simulink model "nms_3Dmodel"  (Simulink 9.3)
settings: Solver=ode15s  StartTime=0.0  StopTime=20  FixedStep=1e-3  RelTol=1e-3  AbsTol=1e-4  EnableMultiTasking=on
InitFcn:
  | runScripts;
undefined symbols (not defined in the file or in its folder): ankle_height, c, c_jointstop, CtrlPar_FP, CtrlPar_FP_R, CtrlPar_LL, CtrlPar_St, CtrlPar_St_R, CtrlPar_Sw, CtrlPar_Sw_R, CtrlPar_theta0, CtrlPar_Tr, CtrlPar_Tr_R, D12_F, D12_S, D12_T, D12z_T, D13_F, D1G_F, D1G_HAT, D1G_S, D1G_T, D1Gy_F, d_fBall, d_fHeel, DeltaThRef, dt, eref, FmaxBFSH, FmaxGAS, FmaxGLU, FmaxHAB, FmaxHAD, FmaxHAM, FmaxHFL, FmaxRF, FmaxSOL, FmaxTA, FmaxVAS, In_F, In_HAT, In_S, In_T, init_a_tgt, init_a_tgtR, Inx_F, Inx_HAT, Inx_S, Inx_T, Iny_F, Iny_HAT, Iny_S, Iny_T, K, k_gn, k_gt, k_pressure, leg_l, LongDelay, LongLoopDelay ... (+137)
libraries: mblibv1 x88, simulink x44, simulink_extras x38
(part 3 of 13)

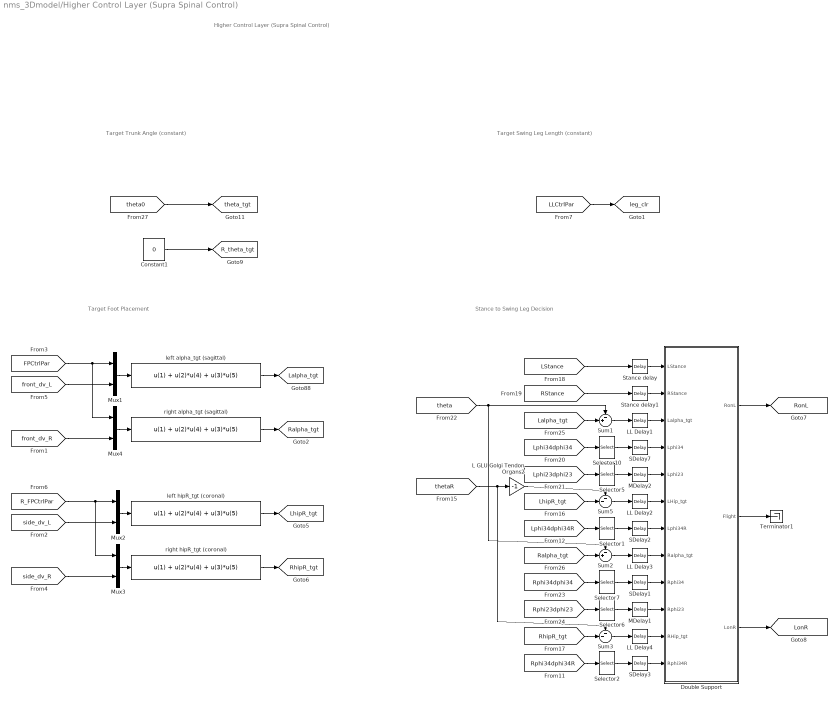
== system nms_3Dmodel/Higher Control Layer (Supra Spinal Control) ==
  note: Target Foot Placement
  note: Target Swing Leg Length
      | (constant)
  note: Stance to Swing Leg Decision
  note: Target Trunk Angle
      | (constant)
  note: Higher Control Layer
      | (Supra Spinal Control)
  Constant1 : Constant  Value=0
  Double Support : Subsystem
  L GLU Golgi Tendon Organs2 : Gain  Gain=-1
  LL Delay1 : TransportDelay  DelayTime=LongLoopDelay/2  InitialOutput=init_a_tgt
  LL Delay2 : TransportDelay  DelayTime=LongLoopDelay/2
  LL Delay3 : TransportDelay  DelayTime=LongLoopDelay/2  InitialOutput=init_a_tgt
  LL Delay4 : TransportDelay  DelayTime=LongLoopDelay/2
  MDelay1 : TransportDelay  DelayTime=MidDelay
  MDelay2 : TransportDelay  DelayTime=MidDelay
  Mux{1..4} (4 alike) : Mux  Inputs=2
  SDelay{1..3,7} (4 alike) : TransportDelay  DelayTime=ShortDelay
  Selector{1..2,5..7,10} (6 alike) : Selector  InputPortWidth=2  IndexOptions=Index vector (dialog)  Indices=1  OutputSizes=1
  Stance delay : TransportDelay  DelayTime=MidDelay
  Stance delay1 : TransportDelay  DelayTime=MidDelay
  Sum1 : Sum  Inputs=-+|
  Sum2 : Sum  Inputs=-+|
  Sum3 : Sum  Inputs=--|
  Sum5 : Sum  Inputs=--|
  Terminator1 : Terminator
  left alpha_tgt (sagittal) : Fcn  Expr=u(1) + u(2)*u(4) + u(3)*u(5)
  left hipR_tgt (coronal) : Fcn  Expr=u(1) + u(2)*u(4) + u(3)*u(5)
  right alpha_tgt (sagittal) : Fcn  Expr=u(1) + u(2)*u(4) + u(3)*u(5)
  right hipR_tgt (coronal) : Fcn  Expr=u(1) + u(2)*u(4) + u(3)*u(5)
  tag scope: Lalpha_tgt=global, LhipR_tgt=global, LonR=global, R_theta_tgt=global, Ralpha_tgt=global, RhipR_tgt=global, RonL=global, leg_clr=global, theta_tgt=global
  wires:
  left alpha_tgt (sagittal)/1 -> [Lalpha_tgt]
  right alpha_tgt (sagittal)/1 -> [Ralpha_tgt]
  left hipR_tgt (coronal)/1 -> [LhipR_tgt]
  right hipR_tgt (coronal)/1 -> [RhipR_tgt]
  [LLCtrlPar] -> [leg_clr]
  [Lphi34dphi34] -> Selector10/1
  [Lphi23dphi23] -> Selector5/1
  Selector10/1 -> SDelay7/1
  Selector5/1 -> MDelay2/1
  [Rphi34dphi34] -> Selector7/1
  [Rphi23dphi23] -> Selector6/1
  Selector7/1 -> SDelay1/1
  Selector6/1 -> MDelay1/1
  Double Support/3(LonR) -> [LonR]
  Stance delay/1 -> Double Support/1(LStance)
  Stance delay1/1 -> Double Support/2(RStance)
  Double Support/1(RonL) -> [RonL]
  [LStance] -> Stance delay/1
  [RStance] -> Stance delay1/1
  Double Support/2(Flight) -> Terminator1/1
  LL Delay1/1 -> Double Support/3(Lalpha_tgt)
  LL Delay3/1 -> Double Support/8(Ralpha_tgt)
  SDelay7/1 -> Double Support/4(Lphi34)
  SDelay1/1 -> Double Support/9(Rphi34)
  MDelay2/1 -> Double Support/5(Lphi23)
  MDelay1/1 -> Double Support/10(Rphi23)
  Sum1/1 -> LL Delay1/1
  [Lalpha_tgt] -> Sum1/2
  [theta] -> Sum1/1, Sum2/1
  [Ralpha_tgt] -> Sum2/2
  Sum2/1 -> LL Delay3/1
  [Lphi34dphi34R] -> Selector1/1
  Selector1/1 -> SDelay2/1
  SDelay2/1 -> Double Support/7(Lphi34R)
  LL Delay2/1 -> Double Support/6(LHip_tgt)
  Sum5/1 -> LL Delay2/1
  [LhipR_tgt] -> Sum5/2
  [thetaR] -> L GLU Golgi Tendon Organs2/1, Sum3/1
  L GLU Golgi Tendon Organs2/1 -> Sum5/1
  [Rphi34dphi34R] -> Selector2/1
  Selector2/1 -> SDelay3/1
  SDelay3/1 -> Double Support/12(Rphi34R)
  LL Delay4/1 -> Double Support/11(RHip_tgt)
  Sum3/1 -> LL Delay4/1
  [RhipR_tgt] -> Sum3/2
  [theta0] -> [theta_tgt]
  Constant1/1 -> [R_theta_tgt]
  Mux1/1 -> left alpha_tgt (sagittal)/1
  [FPCtrlPar] -> Mux4/1, Mux1/1
  [front_dv_L] -> Mux1/2
  Mux4/1 -> right alpha_tgt (sagittal)/1
  [front_dv_R] -> Mux4/2
  Mux2/1 -> left hipR_tgt (coronal)/1
  Mux3/1 -> right hipR_tgt (coronal)/1
  [R_FPCtrlPar] -> Mux3/1, Mux2/1
  [side_dv_L] -> Mux2/2
  [side_dv_R] -> Mux3/2

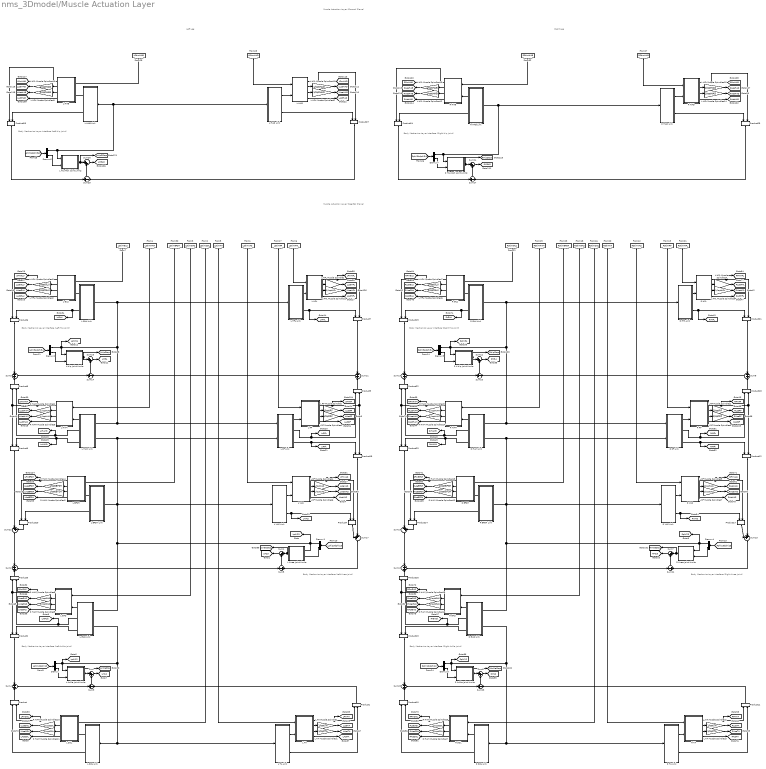
== system nms_3Dmodel/Muscle Actuation Layer ==
  note: Muscle Actuation Layer
      | (Sagittal Plane)
  note: Body Mechanics Layer
      | Interface (Left Hip Joint)
  note: Body Mechanics Layer
      | Interface (Left Knee Joint)
  note: Body Mechanics Layer
      | Interface (Left Ankle Joint)
  note: Body Mechanics Layer
      | Interface (Right Hip Joint)
  note: Body Mechanics Layer
      | Interface (Right Knee Joint)
  note: Body Mechanics Layer
      | Interface (Right Ankle Joint)
  note: Left Leg
  note: Body Mechanics Layer
      | Interface (Left Hip Joint)
  note: Body Mechanics Layer
      | Interface (Right Hip Joint)
  note: Right Leg
  note: Muscle Actuation Layer
      | (Coronal Plane)
  Demux{,1..7} (8 alike) : Demux  Outputs=2
  L Ankle Joint Limits : Subsystem
  L BFSH : Subsystem
  L BFSH Link : Subsystem
  L GAS : Subsystem
  L GAS Link : Subsystem
  L GLU : Subsystem
  L GLU Link : Subsystem
  L HAB : Subsystem
  L HAB Link : Subsystem
  L HAD : Subsystem
  L HAD Link : Subsystem
  L HAM : Subsystem
  L HAM Link : Subsystem
  L HFL : Subsystem
  L HFL Muscle Spindles{,1,4..5} (4 alike) : Gain  Gain=1/loptHFL
  L HFL Muscle Spindles{9..10,12..13} (4 alike) : Gain  Gain=1/loptHAB
  L HFL Muscle Spindles{8,11,14..15} (4 alike) : Gain  Gain=1/loptHAD
  L HFL Muscle Spindles{2..3,6..7} (4 alike) : Gain  Gain=1/loptGLU
  L HFL Link : Subsystem
  L Hip Joint Limits : Subsystem
  L Hip Roll Joint Limits : Subsystem
  L Knee Joint Limits : Subsystem
  L RF : Subsystem
  L RF Muscle Spindles{,1..3} (4 alike) : Gain  Gain=1/loptRF
  L RF Muscle Spindles{4..7} (4 alike) : Gain  Gain=1/loptVAS
  L RF Link : Subsystem
  L SOL : Subsystem
  L SOL Link : Subsystem
  L TA : Subsystem
  L TA Muscle Spindles{,1..3} (4 alike) : Gain  Gain=1/loptTA
  L TA Link : Subsystem
  L VAS : Subsystem
  L VAS Link : Subsystem
  Product{,1..27} (28 alike) : Product  RndMeth=Zero
  R Ankle Joint Limits : Subsystem
  R BFSH : Subsystem
  R BFSH Link : Subsystem
  R GAS : Subsystem
  R GAS Link : Subsystem
  R GLU : Subsystem
  R GLU Link : Subsystem
  R HAB : Subsystem
  R HAB Link : Subsystem
  R HAD : Subsystem
  R HAD Link : Subsystem
  R HAM : Subsystem
  R HAM Muscle Spindles{1,3,6,14} (4 alike) : Gain  Gain=1/loptHAM
  R HAM Muscle Spindles{5,7,10..11} (4 alike) : Gain  Gain=1/loptSOL
  R HAM Muscle Spindles{2,4,12..13} (4 alike) : Gain  Gain=1/loptBFSH
  R HAM Muscle Spindles{8..9,15..16} (4 alike) : Gain  Gain=1/loptGAS
  R HAM Link : Subsystem
  R HFL : Subsystem
  R HFL Link : Subsystem
  R Hip Roll Joint Limits : Subsystem
  R Knee Joint Limits : Subsystem
  R L Hip Joint Limits : Subsystem
  R RF : Subsystem
  R RF Link : Subsystem
  R SOL : Subsystem
  R SOL Link : Subsystem
  R TA : Subsystem
  R TA Link : Subsystem
  R VAS : Subsystem
  R VAS Link : Subsystem
  Sum{,1,6..7,12,16,18,22,24,26} (10 alike) : Sum  Inputs=|++
  Sum{9..10,14,23,25,27} (6 alike) : Sum  Inputs=+-
  Sum{2..4,8,11,15,19..20} (8 alike) : Sum
  Sum13 : Sum  Inputs=++|
  Sum17 : Sum  Inputs=++|
  Sum21 : Sum  Inputs=-+
  Sum5 : Sum  Inputs=-+
  tag scope: LActBFSH=global, LActGAS=global, LActGLU=global, LActHAB=global, LActHAD=global, LActHAM=global, LActHFL=global, LActRF=global, LActSOL=global, LActTA=global, LActVAS=global, LAnkleStop=global, LFmBFSH=global, LFmGAS=global, LFmGLU=global, LFmHAB=global, LFmHAD=global, LFmHAM=global, LFmHFL=global, LFmRF=global, LFmSOL=global, LFmTA=global, LFmVAS=global, LHipRStop=global, LHipStop=global, LKneeStop=global, LLceBFSH=global, LLceGAS=global, LLceGLU=global, LLceHAB=global, LLceHAD=global, LLceHAM=global, LLceHFL=global, LLceRF=global, LLceSOL=global, LLceTA=global, LLceVAS=global, LM12=global, LM23=global, LM34=global, LM34R=global, LVceBFSH=global, LVceGAS=global, LVceGLU=global, LVceHAB=global, LVceHAD=global, LVceHAM=global, LVceHFL=global, LVceRF=global, LVceSOL=global, LVceTA=global, LVceVAS=global, Lphi12=global, Lphi23=global, Lphi34=global, LrGASk=global, LrGLU=global, LrHAMh=global, LrHAMk=global, LrHFL=global, LrRFh=global, LrRFk=global, LrVAS=global, RActBFSH=global, RActGAS=global, RActGLU=global, RActHAB=global, RActHAD=global, RActHAM=global, RActHFL=global, RActRF=global, RActSOL=global, RActTA=global, RActVAS=global, RAnkleStop=global, RFmBFSH=global, RFmGAS=global, RFmGLU=global, RFmHAB=global, RFmHAD=global, RFmHAM=global, RFmHFL=global, RFmRF=global, RFmSOL=global, RFmTA=global, RFmVAS=global, RHipStop=global, RHipStopR=global, RKneeStop=global, RLceBFSH=global, RLceGAS=global, RLceGLU=global, RLceHAB=global, RLceHAD=global, RLceHAM=global, RLceHFL=global, RLceRF=global, RLceSOL=global, RLceTA=global, RLceVAS=global, RM12=global, RM23=global, RM34=global, RM34R=global, RVceBFSH=global, RVceGAS=global, RVceGLU=global, RVceHAB=global, RVceHAD=global, RVceHAM=global, RVceHFL=global, RVceRF=global, RVceSOL=global, RVceTA=global, RVceVAS=global, Rphi12=global, Rphi23=global, Rphi34=global, RrGASk=global, RrGLU=global, RrHAMh=global, RrHAMk=global, RrHFL=global, RrRFh=global, RrRFk=global, RrVAS=global
  wires:
  Demux1/1 -> L Knee Joint Limits/1(phi [rad]), L VAS Link/1(phi23 [rad]), L RF Link/2(phi23 [rad]), L HAM Link/2(phi23 [rad]), L BFSH Link/1(phi23 [rad]), L GAS Link/1(phi23 [rad]), [Lphi23]
  L SOL/1(Fmtc) -> Product/2, [LFmSOL]
  L TA/2(Lce) -> L TA Muscle Spindles/1
  L TA/4(A) -> [LActTA]
  L GAS/1(Fmtc) -> Product2/1, Product3/1, [LFmGAS]
  Demux/1 -> L SOL Link/1(phi12 [rad]), L TA Link/1(phi12 [rad]), L GAS Link/2(phi12 [rad]), L Ankle Joint Limits/1(phi [rad]), [Lphi12]
  [LStimTA] -> L TA/1(STIM)
  [LStimSOL] -> L SOL/1(STIM)
  [LStimHAM] -> L HAM/1(STIM)
  L HAM/1(Fmtc) -> Product9/1, Product8/1, [LFmHAM]
  L HAM/2(Lce) -> R HAM Muscle Spindles1/1
  L HFL/1(Fmtc) -> Product7/2, [LFmHFL]
  L HFL/2(Lce) -> L HFL Muscle Spindles/1
  [LStimHFL] -> L HFL/1(STIM)
  L GLU/1(Fmtc) -> Product6/1, [LFmGLU]
  [LStimGLU] -> L GLU/1(STIM)
  Sum16/1 -> [LM34]
  Demux/2 -> L Ankle Joint Limits/2(dphi [rad/s])
  Sum9/1 -> Sum/2
  Demux1/2 -> L Knee Joint Limits/2(dphi [rad/s])
  L SOL Link/1(lmtc [m]) -> L SOL/2(lmtc [m])
  L TA Link/1(lmtc [m]) -> L TA/2(lmtc [m])
  L GAS Link/3(lever12 [m]) -> Product2/2
  L GAS Link/2(lever23 [m]) -> Product3/2, [LrGASk]
  [LStimGAS] -> L GAS/1(STIM)
  L GAS Link/1(lmtu [m]) -> L GAS/2(lmtc [m])
  L VAS Link/1(lmtu [m]) -> L VAS/2(lmtc [m])
  L HAM Link/1(lmtu [m]) -> L HAM/2(lmtc [m])
  L HAM Link/2(lever34 [m]) -> Product8/2, [LrHAMh]
  L HAM Link/3(lever23 [m]) -> Product9/2, [LrHAMk]
  Product3/1 -> Sum2/2
  Sum3/1 -> Sum14/1
  Sum4/1 -> Sum9/1
  [Lphi12dphi12] -> Demux/1
  [Lphi23dphi23] -> Demux1/1
  [Lphi34dphi34] -> Demux2/1
  Demux2/1 -> L Hip Joint Limits/1(phi [rad]), L HFL Link/1(phi34 [rad]), L GLU Link/1(phi34 [rad]), L RF Link/1(phi34 [rad]), L HAM Link/1(phi34 [rad]), [Lphi34]
  L SOL Link/2(lever [m]) -> Product/1
  Product/1 -> Sum4/2
  Product2/1 -> Sum4/1
  L TA Link/2(lever [m]) -> Product1/2
  Product1/1 -> Sum9/2
  L Ankle Joint Limits/1(M_stop [Nm]) -> Sum/1, [LAnkleStop]
  Sum/1 -> [LM12]
  L SOL/4(A) -> [LActSOL]
  L GAS/4(A) -> [LActGAS]
  L VAS/4(A) -> [LActVAS]
  L VAS/1(Fmtc) -> Product4/2, [LFmVAS]
  Sum1/1 -> [LM23]
  L Knee Joint Limits/1(M_stop [Nm]) -> Sum1/1, [LKneeStop]
  Sum5/1 -> Sum1/2
  L VAS Link/2(lever [m]) -> [LrVAS], Product4/1
  Sum2/1 -> Sum5/1
  L HAM/4(A) -> [LActHAM]
  Product8/1 -> Sum3/2
  Product6/1 -> Sum3/1
  L GLU Link/1(lmtu [m]) -> L GLU/2(lmtc [m])
  L GLU Link/2(lever [m]) -> Product6/2, [LrGLU]
  L GLU/4(A) -> [LActGLU]
  Demux2/2 -> L Hip Joint Limits/2(dphi [rad/s])
  L Hip Joint Limits/1(M_stop [Nm]) -> Sum16/1, [LHipStop]
  Sum14/1 -> Sum16/2
  L HFL Link/1(lmtu [m]) -> L HFL/2(lmtc [m])
  L HFL/4(A) -> [LActHFL]
  L HFL Link/2(lever [m]) -> Product7/1, [LrHFL]
  [LStimVAS] -> L VAS/1(STIM)
  L GLU/2(Lce) -> L HFL Muscle Spindles3/1
  L GLU/3(Vce) -> L HFL Muscle Spindles2/1
  L HAM/3(Vce) -> R HAM Muscle Spindles6/1
  L GAS/3(Vce) -> R HAM Muscle Spindles9/1
  L GAS/2(Lce) -> R HAM Muscle Spindles8/1
  L SOL/2(Lce) -> R HAM Muscle Spindles10/1
  L SOL/3(Vce) -> R HAM Muscle Spindles11/1
  L TA/3(Vce) -> L TA Muscle Spindles1/1
  L VAS/3(Vce) -> L RF Muscle Spindles6/1
  L VAS/2(Lce) -> L RF Muscle Spindles4/1
  L HFL/3(Vce) -> L HFL Muscle Spindles1/1
  L RF/4(A) -> [LActRF]
  L RF/3(Vce) -> L RF Muscle Spindles2/1
  L RF/2(Lce) -> L RF Muscle Spindles/1
  L RF Link/1(lmtu [m]) -> L RF/2(lmtc [m])
  L RF Link/2(lever34 [m]) -> Product5/1, [LrRFh]
  L RF Link/3(lever23 [m]) -> Product15/1, [LrRFk]
  [LStimRF] -> L RF/1(STIM)
  Product7/1 -> Sum11/1
  Product5/1 -> Sum11/2
  Product15/1 -> Sum17/2
  Sum17/1 -> Sum5/2
  Product4/1 -> Sum17/1
  [LStimBFSH] -> L BFSH/1(STIM)
  L BFSH Link/1(lmtu [m]) -> L BFSH/2(lmtc [m])
  L BFSH Link/2(lever [m]) -> Product20/2
  L BFSH/4(A) -> [LActBFSH]
  L BFSH/2(Lce) -> R HAM Muscle Spindles4/1
  L BFSH/3(Vce) -> R HAM Muscle Spindles2/1
  Product20/1 -> Sum22/2
  Sum22/1 -> Sum2/1
  Product9/1 -> Sum22/1
  L HFL Muscle Spindles1/1 -> [LVceHFL]
  L HFL Muscle Spindles2/1 -> [LVceGLU]
  L HFL Muscle Spindles3/1 -> [LLceGLU]
  L RF Muscle Spindles6/1 -> [LVceVAS]
  L RF/1(Fmtc) -> Product5/2, Product15/2, [LFmRF]
  L BFSH/1(Fmtc) -> Product20/1, [LFmBFSH]
  R HAM Muscle Spindles8/1 -> [LLceGAS]
  R HAM Muscle Spindles9/1 -> [LVceGAS]
  R HAM Muscle Spindles10/1 -> [LLceSOL]
  R HAM Muscle Spindles11/1 -> [LVceSOL]
  L TA/1(Fmtc) -> Product1/1, [LFmTA]
  L TA Muscle Spindles1/1 -> [LVceTA]
  L HFL Muscle Spindles/1 -> [LLceHFL]
  R HAM Muscle Spindles1/1 -> [LLceHAM]
  R HAM Muscle Spindles6/1 -> [LVceHAM]
  L RF Muscle Spindles/1 -> [LLceRF]
  L RF Muscle Spindles2/1 -> [LVceRF]
  R HAM Muscle Spindles4/1 -> [LLceBFSH]
  R HAM Muscle Spindles2/1 -> [LVceBFSH]
  L RF Muscle Spindles4/1 -> [LLceVAS]
  L TA Muscle Spindles/1 -> [LLceTA]
  Demux4/1 -> R Knee Joint Limits/1(phi [rad]), R VAS Link/1(phi23 [rad]), R RF Link/2(phi23 [rad]), R HAM Link/2(phi23 [rad]), R BFSH Link/1(phi23 [rad]), R GAS Link/1(phi23 [rad]), [Rphi23]
  R SOL/1(Fmtc) -> Product10/2, [RFmSOL]
  R TA/2(Lce) -> L TA Muscle Spindles2/1
  R TA/4(A) -> [RActTA]
  R GAS/1(Fmtc) -> Product13/1, Product16/1, [RFmGAS]
  Demux3/1 -> R SOL Link/1(phi12 [rad]), R TA Link/1(phi12 [rad]), R GAS Link/2(phi12 [rad]), R Ankle Joint Limits/1(phi [rad]), [Rphi12]
  [RStimTA] -> R TA/1(STIM)
  [RStimSOL] -> R SOL/1(STIM)
  [RStimHAM] -> R HAM/1(STIM)
  R HAM/1(Fmtc) -> Product23/1, Product22/1, [RFmHAM]
  R HAM/2(Lce) -> R HAM Muscle Spindles3/1
  R HFL/1(Fmtc) -> Product21/2, [RFmHFL]
  R HFL/2(Lce) -> L HFL Muscle Spindles4/1
  [RStimHFL] -> R HFL/1(STIM)
  R GLU/1(Fmtc) -> Product19/1, [RFmGLU]
  [RStimGLU] -> R GLU/1(STIM)
  Sum12/1 -> [RM34]
  Demux3/2 -> R Ankle Joint Limits/2(dphi [rad/s])
  Sum23/1 -> Sum6/2
  Demux4/2 -> R Knee Joint Limits/2(dphi [rad/s])
  R SOL Link/1(lmtc [m]) -> R SOL/2(lmtc [m])
  R TA Link/1(lmtc [m]) -> R TA/2(lmtc [m])
  R GAS Link/3(lever12 [m]) -> Product13/2
  R GAS Link/2(lever23 [m]) -> Product16/2, [RrGASk]
  [RStimGAS] -> R GAS/1(STIM)
  R GAS Link/1(lmtu [m]) -> R GAS/2(lmtc [m])
  R VAS Link/1(lmtu [m]) -> R VAS/2(lmtc [m])
  R HAM Link/1(lmtu [m]) -> R HAM/2(lmtc [m])
  R HAM Link/2(lever34 [m]) -> Product22/2, [RrHAMh]
  R HAM Link/3(lever23 [m]) -> Product23/2, [RrHAMk]
  Product16/1 -> Sum15/2
  Sum19/1 -> Sum10/1
  Sum20/1 -> Sum23/1
  [Rphi12dphi12] -> Demux3/1
  [Rphi23dphi23] -> Demux4/1
  [Rphi34dphi34] -> Demux5/1
  Demux5/1 -> R L Hip Joint Limits/1(phi [rad]), R HFL Link/1(phi34 [rad]), R GLU Link/1(phi34 [rad]), R RF Link/1(phi34 [rad]), R HAM Link/1(phi34 [rad]), [Rphi34]
  R SOL Link/2(lever [m]) -> Product10/1
  Product10/1 -> Sum20/2
  Product13/1 -> Sum20/1
  R TA Link/2(lever [m]) -> Product11/2
  Product11/1 -> Sum23/2
  R Ankle Joint Limits/1(M_stop [Nm]) -> Sum6/1, [RAnkleStop]
  Sum6/1 -> [RM12]
  R SOL/4(A) -> [RActSOL]
  R GAS/4(A) -> [RActGAS]
  R VAS/4(A) -> [RActVAS]
  R VAS/1(Fmtc) -> Product17/2, [RFmVAS]
  Sum7/1 -> [RM23]
  R Knee Joint Limits/1(M_stop [Nm]) -> Sum7/1, [RKneeStop]
  Sum21/1 -> Sum7/2
  R VAS Link/2(lever [m]) -> [RrVAS], Product17/1
  Sum15/1 -> Sum21/1
  R HAM/4(A) -> [RActHAM]
  Product22/1 -> Sum19/2
  Product19/1 -> Sum19/1
  R GLU Link/1(lmtu [m]) -> R GLU/2(lmtc [m])
  R GLU Link/2(lever [m]) -> Product19/2, [RrGLU]
  R GLU/4(A) -> [RActGLU]
  Demux5/2 -> R L Hip Joint Limits/2(dphi [rad/s])
  R L Hip Joint Limits/1(M_stop [Nm]) -> Sum12/1, [RHipStop]
  Sum10/1 -> Sum12/2
  R HFL Link/1(lmtu [m]) -> R HFL/2(lmtc [m])
  R HFL/4(A) -> [RActHFL]
  R HFL Link/2(lever [m]) -> Product21/1, [RrHFL]
  [RStimVAS] -> R VAS/1(STIM)
  R GLU/2(Lce) -> L HFL Muscle Spindles7/1
  R GLU/3(Vce) -> L HFL Muscle Spindles6/1
  R HAM/3(Vce) -> R HAM Muscle Spindles14/1
  R GAS/3(Vce) -> R HAM Muscle Spindles16/1
  R GAS/2(Lce) -> R HAM Muscle Spindles15/1
  R SOL/2(Lce) -> R HAM Muscle Spindles5/1
  R SOL/3(Vce) -> R HAM Muscle Spindles7/1
  R TA/3(Vce) -> L TA Muscle Spindles3/1
  R VAS/3(Vce) -> L RF Muscle Spindles7/1
  R VAS/2(Lce) -> L RF Muscle Spindles5/1
  R HFL/3(Vce) -> L HFL Muscle Spindles5/1
  R RF/4(A) -> [RActRF]
  R RF/3(Vce) -> L RF Muscle Spindles3/1
  R RF/2(Lce) -> L RF Muscle Spindles1/1
  R RF Link/1(lmtu [m]) -> R RF/2(lmtc [m])
  R RF Link/2(lever34 [m]) -> Product18/1, [RrRFh]
  R RF Link/3(lever23 [m]) -> Product12/1, [RrRFk]
  [RStimRF] -> R RF/1(STIM)
  Sum8/1 -> Sum10/2
  Product21/1 -> Sum8/1
  Product18/1 -> Sum8/2
  Product12/1 -> Sum13/2
  Sum13/1 -> Sum21/2
  Product17/1 -> Sum13/1
  [RStimBFSH] -> R BFSH/1(STIM)
  R BFSH Link/1(lmtu [m]) -> R BFSH/2(lmtc [m])
  R BFSH Link/2(lever [m]) -> Product14/2
  R BFSH/4(A) -> [RActBFSH]
  R BFSH/2(Lce) -> R HAM Muscle Spindles13/1
  R BFSH/3(Vce) -> R HAM Muscle Spindles12/1
  Product14/1 -> Sum18/2
  Sum18/1 -> Sum15/1
  Product23/1 -> Sum18/1
  L HFL Muscle Spindles5/1 -> [RVceHFL]
  L HFL Muscle Spindles6/1 -> [RVceGLU]
  L HFL Muscle Spindles7/1 -> [RLceGLU]
  L RF Muscle Spindles7/1 -> [RVceVAS]
  R RF/1(Fmtc) -> Product18/2, Product12/2, [RFmRF]
  R BFSH/1(Fmtc) -> Product14/1, [RFmBFSH]
  R HAM Muscle Spindles15/1 -> [RLceGAS]
  R HAM Muscle Spindles16/1 -> [RVceGAS]
  R HAM Muscle Spindles5/1 -> [RLceSOL]
  R HAM Muscle Spindles7/1 -> [RVceSOL]
  R TA/1(Fmtc) -> Product11/1, [RFmTA]
  L TA Muscle Spindles3/1 -> [RVceTA]
  L HFL Muscle Spindles4/1 -> [RLceHFL]
  R HAM Muscle Spindles3/1 -> [RLceHAM]
  R HAM Muscle Spindles14/1 -> [RVceHAM]
  L RF Muscle Spindles1/1 -> [RLceRF]
  L RF Muscle Spindles3/1 -> [RVceRF]
  R HAM Muscle Spindles13/1 -> [RLceBFSH]
  R HAM Muscle Spindles12/1 -> [RVceBFSH]
  L RF Muscle Spindles5/1 -> [RLceVAS]
  L TA Muscle Spindles2/1 -> [RLceTA]
  Sum11/1 -> Sum14/2
  [LStimHAD] -> L HAD/1(STIM)
  [LStimHAB] -> L HAB/1(STIM)
  Sum26/1 -> [LM34R]
  [Lphi34dphi34R] -> Demux6/1
  Demux6/1 -> L HAB Link/1(phi34R [rad]), L HAD Link/1(phi34R [rad]), L Hip Roll Joint Limits/1(phi [rad])
  Product26/1 -> Sum25/1
  L HAB Link/1(lmtu [m]) -> L HAB/2(lmtc [m])
  L HAB Link/2(lever [m]) -> Product26/2
  Demux6/2 -> L Hip Roll Joint Limits/2(dphi [rad/s])
  L Hip Roll Joint Limits/1(M_stop [Nm]) -> Sum26/1, [LHipRStop]
  Sum25/1 -> Sum26/2
  Product27/1 -> Sum25/2
  L HAD Link/1(lmtu [m]) -> L HAD/2(lmtc [m])
  L HAD Link/2(lever [m]) -> Product27/1
  [RStimHAD] -> R HAD/1(STIM)
  Sum24/1 -> [RM34R]
  [Rphi34dphi34R] -> Demux7/1
  Demux7/1 -> R HAD Link/1(phi34R [rad]), R HAB Link/1(phi34R [rad]), R Hip Roll Joint Limits/1(phi [rad])
  Product24/1 -> Sum27/1
  R HAB Link/1(lmtu [m]) -> R HAB/2(lmtc [m])
  R HAB Link/2(lever [m]) -> Product24/2
  Demux7/2 -> R Hip Roll Joint Limits/2(dphi [rad/s])
  R Hip Roll Joint Limits/1(M_stop [Nm]) -> Sum24/1, [RHipStopR]
  Sum27/1 -> Sum24/2
  Product25/1 -> Sum27/2
  R HAD Link/1(lmtu [m]) -> R HAD/2(lmtc [m])
  R HAD Link/2(lever [m]) -> Product25/1
  [RStimHAB] -> R HAB/1(STIM)
  L HAB/4(A) -> [LActHAB]
  L HAB/2(Lce) -> L HFL Muscle Spindles10/1
  L HAB/3(Vce) -> L HFL Muscle Spindles9/1
  L HFL Muscle Spindles9/1 -> [LVceHAB]
  L HFL Muscle Spindles10/1 -> [LLceHAB]
  L HAB/1(Fmtc) -> Product26/1, [LFmHAB]
  L HFL Muscle Spindles8/1 -> [LVceHAD]
  L HFL Muscle Spindles11/1 -> [LLceHAD]
  L HAD/2(Lce) -> L HFL Muscle Spindles11/1
  L HAD/3(Vce) -> L HFL Muscle Spindles8/1
  L HAD/4(A) -> [LActHAD]
  L HAD/1(Fmtc) -> [LFmHAD], Product27/2
  R HAB/4(A) -> [RActHAB]
  R HAB/2(Lce) -> L HFL Muscle Spindles13/1
  R HAB/3(Vce) -> L HFL Muscle Spindles12/1
  L HFL Muscle Spindles12/1 -> [RVceHAB]
  L HFL Muscle Spindles13/1 -> [RLceHAB]
  R HAB/1(Fmtc) -> [RFmHAB], Product24/1
  L HFL Muscle Spindles14/1 -> [RVceHAD]
  L HFL Muscle Spindles15/1 -> [RLceHAD]
  R HAD/2(Lce) -> L HFL Muscle Spindles15/1
  R HAD/3(Vce) -> L HFL Muscle Spindles14/1
  R HAD/4(A) -> [RActHAD]
  R HAD/1(Fmtc) -> [RFmHAD], Product25/2

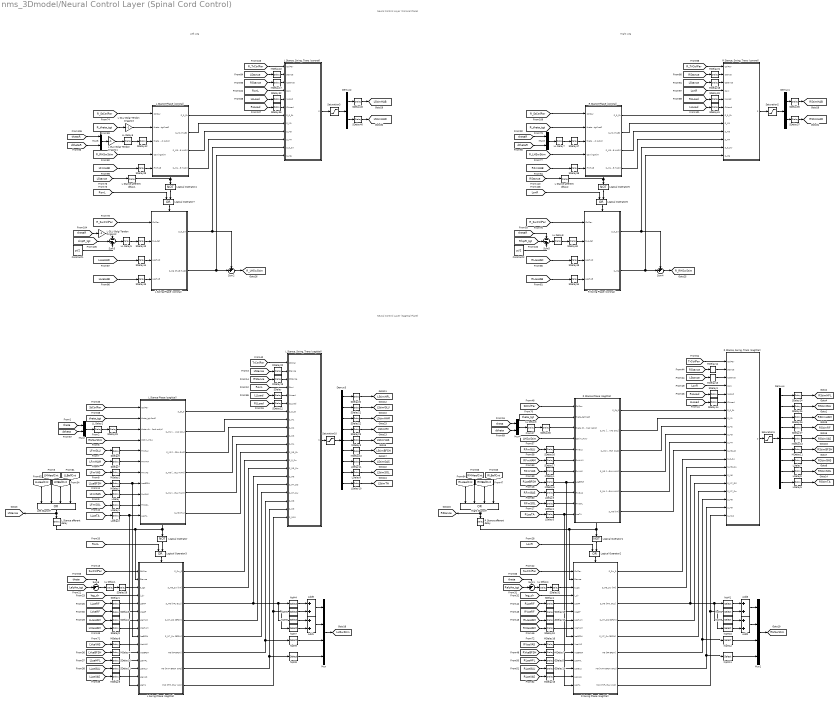
== system nms_3Dmodel/Neural Control Layer (Spinal Cord Control) ==
  note: Neural Control Layer
      | (Sagittal Plane)
  note: Neural Control Layer
      | (Coronal Plane)
  note: Right Leg
  note: Left Leg
  Add{1..3,9} (4 alike) : Sum  Inputs=2
  Constant1 : Constant  Value=pi/2
  Constant2 : Constant  Value=pi/2
  Demux1 : Demux  Outputs=2
  Demux2 : Demux  Outputs=2
  Demux3 : Demux  Outputs=9
  Demux4 : Demux  Outputs=9
  L GLU Golgi Tendon Organs1 : Gain  Gain=-1
  L GLU Golgi Tendon Organs2 : Gain  Gain=-1
  L GLU Golgi Tendon Organs3 : Gain  Gain=-1
  L Stance afferent delay : TransportDelay  DelayTime=MidDelay
  L Stance afferent delay1 : TransportDelay  DelayTime=MidDelay
  L Stance afferent delay2 : TransportDelay  DelayTime=MidDelay
  L Stance Phase (coronal) : Subsystem  TreatAsAtomicUnit=on
  L Stance Phase (sagittal) : Subsystem  TreatAsAtomicUnit=on
  "L Stance, Swing, Trans (coronal)" : Subsystem  TreatAsAtomicUnit=on
  "L Stance, Swing, Trans (sagittal)" : Subsystem
  L Swing Phase (coronal) : Subsystem  TreatAsAtomicUnit=on
  L Swing Phase (sagittal) : Subsystem  TreatAsAtomicUnit=on
  LDelay{,1,3..4} (4 alike) : TransportDelay  DelayTime=LongDelay
  LDelay10 : TransportDelay  DelayTime=LongDelay  InitialOutput=St_PreSTA
  LDelay11 : TransportDelay  DelayTime=LongDelay  InitialOutput=St_PreSGAS
  LDelay2 : TransportDelay  DelayTime=LongDelay  InitialOutput=1
  LDelay5 : TransportDelay  DelayTime=LongDelay  InitialOutput=1
  LDelay6 : TransportDelay  DelayTime=LongDelay  InitialOutput=Sw_PreSTA
  LDelay7 : TransportDelay  DelayTime=LongDelay  InitialOutput=Sw_PreSGAS
  LDelay8 : TransportDelay  DelayTime=LongDelay  InitialOutput=Sw_PreSSOL
  LDelay9 : TransportDelay  DelayTime=LongDelay  InitialOutput=St_PreSSOL
  LL Delay1 : TransportDelay  DelayTime=LongLoopDelay/2  InitialOutput=init_a_tgt
  LL Delay{2..3,6..7} (4 alike) : TransportDelay  DelayTime=LongLoopDelay/2
  LL Delay4 : TransportDelay  DelayTime=LongLoopDelay/2  InitialOutput=init_a_tgt
  LL Delay5 : TransportDelay  DelayTime=LongLoopDelay/2  InitialOutput=init_a_tgtR
  LL Delay8 : TransportDelay  DelayTime=LongLoopDelay/2  InitialOutput=init_a_tgtR
  Left Stance? : Logic  Operator=OR  Inputs=4  AllPortsSameDT=off
  Logical Operator{,1,4..5} (4 alike) : Logic  Operator=NOT  AllPortsSameDT=off  OutDataTypeStr=boolean
  Logical Operator{2..3,6..7} (4 alike) : Logic  Operator=OR  AllPortsSameDT=off  OutDataTypeStr=boolean
  MDelay{1..2,4,7..8,13..14,16..22} (14 alike) : TransportDelay  DelayTime=MidDelay
  MDelay10 : TransportDelay  DelayTime=MidDelay  InitialOutput=St_PreSBFSH
  MDelay11 : TransportDelay  DelayTime=MidDelay  InitialOutput=Sw_PreSBFSH
  MDelay12 : TransportDelay  DelayTime=MidDelay  InitialOutput=Sw_PreSVAS
  MDelay{3,5..6,15} (4 alike) : TransportDelay  DelayTime=MidDelay  InitialOutput=1
  MDelay9 : TransportDelay  DelayTime=MidDelay  InitialOutput=St_PreSVAS
  Mux : Mux
  Mux1 : Mux
  Mux{2..5} (4 alike) : Mux  Inputs=2
  R Stance afferent delay : TransportDelay  DelayTime=MidDelay
  R Stance Phase (coronal) : Subsystem  TreatAsAtomicUnit=on
  R Stance Phase (sagittal) : Subsystem  TreatAsAtomicUnit=on
  "R Stance, Swing, Trans (coronal)" : Subsystem  TreatAsAtomicUnit=on
  "R Stance, Swing, Trans (sagittal)" : Subsystem
  R Swing Phase (coronal) : Subsystem  TreatAsAtomicUnit=on
  R Swing Phase (sagittal) : Subsystem  TreatAsAtomicUnit=on
  Right Stance? : Logic  Operator=OR  Inputs=4  AllPortsSameDT=off
  SDelay{,3,6..9,12,14,16..19,29..30,32..33,36,38..39,41..42,47} (22 alike) : TransportDelay  DelayTime=ShortDelay
  SDelay{1..2,4..5,10..11,13,15,34,44..45,49} (12 alike) : TransportDelay  DelayTime=ShortDelay  InitialOutput=1
  SDelay20 : TransportDelay  DelayTime=ShortDelay  InitialOutput=St_PreSHFL
  SDelay21 : TransportDelay  DelayTime=ShortDelay  InitialOutput=St_PreSGLU
  SDelay22 : TransportDelay  DelayTime=ShortDelay  InitialOutput=St_PreSHAM
  SDelay23 : TransportDelay  DelayTime=ShortDelay  InitialOutput=St_PreSRF
  SDelay24 : TransportDelay  DelayTime=ShortDelay  InitialOutput=Sw_PreSHFL
  SDelay25 : TransportDelay  DelayTime=ShortDelay  InitialOutput=Sw_PreSGLU
  SDelay26 : TransportDelay  DelayTime=ShortDelay  InitialOutput=Sw_PreSHAM
  SDelay27 : TransportDelay  DelayTime=ShortDelay  InitialOutput=Sw_PreSRF
  SDelay28 : TransportDelay  DelayTime=ShortDelay  InitialOutput=init_a_tgt
  SDelay31 : TransportDelay  DelayTime=ShortDelay  InitialOutput=init_a_tgt
  SDelay35 : TransportDelay  DelayTime=ShortDelay  InitialOutput=Sw_PreS_HAB
  SDelay37 : TransportDelay  DelayTime=ShortDelay  InitialOutput=Sw_PreS_HAD
  SDelay40 : TransportDelay  DelayTime=ShortDelay  InitialOutput=St_PreS_HAD
  SDelay43 : TransportDelay  DelayTime=ShortDelay  InitialOutput=init_a_tgtR
  SDelay46 : TransportDelay  DelayTime=ShortDelay  InitialOutput=St_PreS_HAB
  SDelay48 : TransportDelay  DelayTime=ShortDelay  InitialOutput=init_a_tgtR
  Saturation{1..3,10} (4 alike) : Saturate  UpperLimit=1  LowerLimit=0.01  ZeroCross=off
  Sum1 : Sum  Inputs=-+|
  Sum2 : Sum  Inputs=++|
  Sum3 : Sum  Inputs=--+
  Sum4 : Sum  Inputs=++|
  Sum5 : Sum  Inputs=--+
  Sum6 : Sum  Inputs=-+|
  hipM{1,4,9,12} (4 alike) : Selector  InputPortWidth=2  IndexOptions=Index vector (dialog)  Indices=1  OutputSizes=1
  hipM10 : Selector  InputPortWidth=3  IndexOptions=Index vector (dialog)  Indices=2  OutputSizes=1
  hipM{2,5,8,11} (4 alike) : Selector  InputPortWidth=3  IndexOptions=Index vector (dialog)  Indices=1  OutputSizes=1
  hipM3 : Selector  InputPortWidth=2  IndexOptions=Index vector (dialog)  Indices=2  OutputSizes=1
  hipM6 : Selector  InputPortWidth=2  IndexOptions=Index vector (dialog)  Indices=2  OutputSizes=1
  hipM7 : Selector  InputPortWidth=3  IndexOptions=Index vector (dialog)  Indices=2  OutputSizes=1
  tag scope: LHSwStim=global, LStance=global, LStimBFSH=global, LStimGAS=global, LStimGLU=global, LStimHAB=global, LStimHAD=global, LStimHAM=global, LStimHFL=global, LStimRF=global, LStimSOL=global, LStimTA=global, LStimVAS=global, RHSwStim=global, RStance=global, RStimBFSH=global, RStimGAS=global, RStimGLU=global, RStimHAB=global, RStimHAD=global, RStimHAM=global, RStimHFL=global, RStimRF=global, RStimSOL=global, RStimTA=global, RStimVAS=global, R_LHSwStim=global, R_RHSwStim=global
  wires:
  [LLLoad] -> SDelay/1
  Left Stance?/1 -> L Stance afferent delay/1, [LStance]
  [StCtrlPar] -> L Stance Phase (sagittal)/1(CtrlPar)
  [RHSwStim] -> L Stance Phase (sagittal)/4(CStim_HSw)
  [LFmGLU] -> SDelay6/1
  SDelay6/1 -> L Stance Phase (sagittal)/5(FmGLU)
  [LFmHAM] -> SDelay7/1
  SDelay7/1 -> L Stance Phase (sagittal)/6(FmHAM)
  [LFmVAS] -> MDelay2/1
  MDelay2/1 -> L Stance Phase (sagittal)/7(FmVAS)
  [LLceBFSH] -> MDelay3/1
  MDelay3/1 -> L Stance Phase (sagittal)/8(LceBFSH), L Swing Phase (sagittal)/9(lceBFSH)
  [LFmGAS] -> LDelay/1
  LDelay/1 -> L Stance Phase (sagittal)/9(FmGAS)
  [LFmSOL] -> LDelay1/1
  LDelay1/1 -> L Stance Phase (sagittal)/10(FmSOL)
  [LLceTA] -> LDelay2/1
  LDelay2/1 -> L Stance Phase (sagittal)/11(LceTA), L Swing Phase (sagittal)/15(LceTA)
  [SwCtrlPar] -> L Swing Phase (sagittal)/1(CtrlPar)
  L Stance afferent delay/1 -> L Stance Phase (sagittal)/Enable, Logical Operator/1, L Swing Phase (sagittal)/2(Stance)
  Logical Operator/1 -> Logical Operator3/2
  Logical Operator3/1 -> L Swing Phase (sagittal)/Enable
  [RonL] -> Logical Operator3/1
  [leg_clr] -> L Swing Phase (sagittal)/4(l_clr)
  [LLceRF] -> SDelay1/1
  SDelay1/1 -> L Swing Phase (sagittal)/5(LceRF)
  [LLceHAM] -> SDelay2/1
  SDelay2/1 -> L Swing Phase (sagittal)/7(LceHAM)
  [LVceRF] -> SDelay8/1
  SDelay8/1 -> L Swing Phase (sagittal)/6(VceRF)
  [LVceHAM] -> SDelay9/1
  SDelay9/1 -> L Swing Phase (sagittal)/8(VceHAM)
  [LVceBFSH] -> MDelay4/1
  MDelay4/1 -> L Swing Phase (sagittal)/11(VceBFSH)
  SDelay10/1 -> L Swing Phase (sagittal)/12(LceHFL)
  SDelay11/1 -> L Swing Phase (sagittal)/13(LceGLU)
  MDelay5/1 -> L Swing Phase (sagittal)/14(LceVAS)
  [TrCtrlPar] -> "L Stance, Swing, Trans (sagittal)"/1(CtrlPar)
  [RLLoad] -> SDelay12/1
  Demux3/1 -> SDelay20/1
  Demux3/2 -> SDelay21/1
  Demux3/3 -> SDelay22/1
  Saturation10/1 -> Demux3/1
  Demux3/7 -> LDelay11/1
  Demux3/8 -> LDelay9/1
  Demux3/9 -> LDelay10/1
  Demux3/4 -> SDelay23/1
  Demux3/5 -> MDelay9/1
  Demux3/6 -> MDelay10/1
  "L Stance, Swing, Trans (sagittal)"/1(S) -> Saturation10/1
  [RonL] -> "L Stance, Swing, Trans (sagittal)"/4(ConI)
  [LStance] -> MDelay20/1
  [RStance] -> MDelay19/1
  Right Stance?/1 -> R Stance afferent delay/1, [RStance]
  [StCtrlPar] -> R Stance Phase (sagittal)/1(CtrlPar)
  [RLLoad] -> SDelay3/1
  [LHSwStim] -> R Stance Phase (sagittal)/4(CStim_HSw)
  [RFmGLU] -> SDelay16/1
  SDelay16/1 -> R Stance Phase (sagittal)/5(FmGLU)
  [RFmHAM] -> SDelay17/1
  SDelay17/1 -> R Stance Phase (sagittal)/6(FmHAM)
  [RFmVAS] -> MDelay1/1
  MDelay1/1 -> R Stance Phase (sagittal)/7(FmVAS)
  [RLceBFSH] -> MDelay6/1
  MDelay6/1 -> R Stance Phase (sagittal)/8(LceBFSH), R Swing Phase (sagittal)/9(lceBFSH)
  [RFmGAS] -> LDelay3/1
  LDelay3/1 -> R Stance Phase (sagittal)/9(FmGAS)
  [RFmSOL] -> LDelay4/1
  LDelay4/1 -> R Stance Phase (sagittal)/10(FmSOL)
  [RLceTA] -> LDelay5/1
  LDelay5/1 -> R Stance Phase (sagittal)/11(LceTA), R Swing Phase (sagittal)/15(LceTA)
  [SwCtrlPar] -> R Swing Phase (sagittal)/1(CtrlPar)
  R Stance afferent delay/1 -> Logical Operator1/1, R Stance Phase (sagittal)/Enable, R Swing Phase (sagittal)/2(Stance)
  Logical Operator1/1 -> Logical Operator2/2
  Logical Operator2/1 -> R Swing Phase (sagittal)/Enable
  [LonR] -> Logical Operator2/1
  [leg_clr] -> R Swing Phase (sagittal)/4(l_clr)
  [RLceRF] -> SDelay4/1
  SDelay4/1 -> R Swing Phase (sagittal)/5(LceRF)
  [RLceHAM] -> SDelay15/1
  SDelay15/1 -> R Swing Phase (sagittal)/7(LceHAM)
  [RVceRF] -> SDelay18/1
  SDelay18/1 -> R Swing Phase (sagittal)/6(VceRF)
  [RVceHAM] -> SDelay19/1
  SDelay19/1 -> R Swing Phase (sagittal)/8(VceHAM)
  [RVceBFSH] -> MDelay7/1
  MDelay7/1 -> R Swing Phase (sagittal)/11(VceBFSH)
  SDelay5/1 -> R Swing Phase (sagittal)/12(LceHFL)
  SDelay13/1 -> R Swing Phase (sagittal)/13(LceGLU)
  MDelay15/1 -> R Swing Phase (sagittal)/14(LceVAS)
  [TrCtrlPar] -> "R Stance, Swing, Trans (sagittal)"/1(CtrlPar)
  SDelay14/1 -> "R Stance, Swing, Trans (sagittal)"/6(CLLoad)
  [LLLoad] -> SDelay14/1
  Saturation1/1 -> Demux4/1
  [LonR] -> "R Stance, Swing, Trans (sagittal)"/4(ConI)
  [RStance] -> MDelay14/1
  [LStance] -> MDelay13/1
  [LLHeelCnt] -> Left Stance?/1
  [LMHeelCnt] -> Left Stance?/2
  [LMBallCnt] -> Left Stance?/3
  [LLBallCnt] -> Left Stance?/4
  [RLHeelCnt] -> Right Stance?/1
  [RMHeelCnt] -> Right Stance?/2
  [RMBallCnt] -> Right Stance?/3
  [RLBallCnt] -> Right Stance?/4
  SDelay12/1 -> "L Stance, Swing, Trans (sagittal)"/6(CLLoad)
  SDelay20/1 -> [LStimHFL]
  SDelay21/1 -> [LStimGLU]
  SDelay22/1 -> [LStimHAM]
  SDelay23/1 -> [LStimRF]
  MDelay9/1 -> [LStimVAS]
  MDelay10/1 -> [LStimBFSH]
  LDelay11/1 -> [LStimGAS]
  LDelay9/1 -> [LStimSOL]
  LDelay10/1 -> [LStimTA]
  Demux4/1 -> SDelay24/1
  Demux4/2 -> SDelay25/1
  Demux4/3 -> SDelay26/1
  Demux4/7 -> LDelay7/1
  Demux4/8 -> LDelay8/1
  Demux4/9 -> LDelay6/1
  Demux4/4 -> SDelay27/1
  Demux4/5 -> MDelay12/1
  Demux4/6 -> MDelay11/1
  SDelay24/1 -> [RStimHFL]
  SDelay25/1 -> [RStimGLU]
  SDelay26/1 -> [RStimHAM]
  SDelay27/1 -> [RStimRF]
  MDelay12/1 -> [RStimVAS]
  MDelay11/1 -> [RStimBFSH]
  LDelay7/1 -> [RStimGAS]
  LDelay8/1 -> [RStimSOL]
  LDelay6/1 -> [RStimTA]
  [Lalpha_tgt] -> Sum6/2
  [theta] -> Sum6/1
  [Ralpha_tgt] -> Sum1/2
  [theta] -> Sum1/1
  MDelay20/1 -> "L Stance, Swing, Trans (sagittal)"/2(Stance)
  MDelay19/1 -> "L Stance, Swing, Trans (sagittal)"/3(CStance)
  MDelay14/1 -> "R Stance, Swing, Trans (sagittal)"/2(Stance)
  MDelay13/1 -> "R Stance, Swing, Trans (sagittal)"/3(CStance)
  [LLceHFL] -> SDelay10/1
  [LLceGLU] -> SDelay11/1
  [LLceVAS] -> MDelay5/1
  [RLceHFL] -> SDelay5/1
  [RLceGLU] -> SDelay13/1
  [RLceVAS] -> MDelay15/1
  LL Delay1/1 -> SDelay28/1
  Sum6/1 -> LL Delay1/1
  SDelay28/1 -> L Swing Phase (sagittal)/3(a_tgt)
  L Stance Phase (sagittal)/1(S_St_0) -> "L Stance, Swing, Trans (sagittal)"/7(S_0_St)
  L Swing Phase (sagittal)/1(S_Sw_0) -> "L Stance, Swing, Trans (sagittal)"/13(S_0_Sw)
  R Stance Phase (sagittal)/1(S_St_0) -> "R Stance, Swing, Trans (sagittal)"/7(S_0_St)
  L Stance Phase (sagittal)/2(S_M1 [GLU VAS SOL]) -> "L Stance, Swing, Trans (sagittal)"/8(S_M1)
  L Stance Phase (sagittal)/3(S_M2 [HAM VAS BFSH GAS]) -> "L Stance, Swing, Trans (sagittal)"/9(S_M2)
  L Stance Phase (sagittal)/6(S_M5 [TA]) -> "L Stance, Swing, Trans (sagittal)"/12(S_M5_St)
  R Stance Phase (sagittal)/2(S_M1 [GLU VAS SOL]) -> "R Stance, Swing, Trans (sagittal)"/8(S_M1)
  R Stance Phase (sagittal)/3(S_M2 [HAM VAS BFSH GAS]) -> "R Stance, Swing, Trans (sagittal)"/9(S_M2)
  R Stance Phase (sagittal)/6(S_M5 [TA]) -> "R Stance, Swing, Trans (sagittal)"/12(S_M5_St)
  [theta] -> Mux2/1
  [dtheta] -> Mux2/2
  [theta_tgt] -> L Stance Phase (sagittal)/2(theta_tgt [rad])
  SDelay/1 -> "L Stance, Swing, Trans (sagittal)"/5(ILLoad)
  [theta] -> Mux4/1
  [dtheta] -> Mux4/2
  [theta_tgt] -> R Stance Phase (sagittal)/2(theta_tgt [rad])
  L Stance Phase (sagittal)/4(S_M3 [HFL GLU HAM]) -> "L Stance, Swing, Trans (sagittal)"/10(S_M3)
  R Stance Phase (sagittal)/4(S_M3 [HFL GLU HAM]) -> "R Stance, Swing, Trans (sagittal)"/10(S_M3)
  SDelay3/1 -> "R Stance, Swing, Trans (sagittal)"/5(ILLoad)
  LL Delay2/1 -> SDelay29/1
  Mux2/1 -> LL Delay2/1
  SDelay29/1 -> L Stance Phase (sagittal)/3(theta dtheta [rad rad/s])
  LL Delay3/1 -> SDelay30/1
  Mux4/1 -> LL Delay3/1
  SDelay30/1 -> R Stance Phase (sagittal)/3(theta dtheta [rad rad/s])
  R Stance Phase (sagittal)/5(S_M4 [HFL GLU HAM]) -> "R Stance, Swing, Trans (sagittal)"/11(S_M4)
  L Stance Phase (sagittal)/5(S_M4 [HFL GLU HAM]) -> "L Stance, Swing, Trans (sagittal)"/11(S_M4)
  L Swing Phase (sagittal)/2(S_M5_Sw [TA]) -> "L Stance, Swing, Trans (sagittal)"/14(S_M5_Sw)
  L Swing Phase (sagittal)/3(S_M6 [HFL GLU]) -> "L Stance, Swing, Trans (sagittal)"/15(S_M6), hipM6/1, hipM4/1
  L Swing Phase (sagittal)/4(S_M7_DS [BFSH]) -> "L Stance, Swing, Trans (sagittal)"/16(S_M7_DS)
  L Swing Phase (sagittal)/5(S_M7_Sw [BFSH]) -> "L Stance, Swing, Trans (sagittal)"/17(S_M7_Sw)
  L Swing Phase (sagittal)/6(M8 [RF BFSH]) -> "L Stance, Swing, Trans (sagittal)"/18(S_M8), hipM9/1
  L Swing Phase (sagittal)/7(M9 [HAM BFSH GAS]) -> "L Stance, Swing, Trans (sagittal)"/19(S_M9), hipM8/1
  L Swing Phase (sagittal)/8(M10 [HFL GLU VAS]) -> "L Stance, Swing, Trans (sagittal)"/20(S_M10), hipM5/1, hipM7/1
  Mux/1 -> [LHSwStim]
  hipM4/1 -> Add9/1
  hipM5/1 -> Add9/2
  Add9/1 -> Mux/1
  hipM6/1 -> Add1/1
  hipM7/1 -> Add1/2
  Add1/1 -> Mux/2
  hipM9/1 -> Mux/3
  hipM8/1 -> Mux/4
  "R Stance, Swing, Trans (sagittal)"/1(S) -> Saturation1/1
  R Swing Phase (sagittal)/1(S_Sw_0) -> "R Stance, Swing, Trans (sagittal)"/13(S_0_Sw)
  R Swing Phase (sagittal)/2(S_M5_Sw [TA]) -> "R Stance, Swing, Trans (sagittal)"/14(S_M5_Sw)
  R Swing Phase (sagittal)/3(S_M6 [HFL GLU]) -> hipM3/1, hipM1/1, "R Stance, Swing, Trans (sagittal)"/15(S_M6)
  R Swing Phase (sagittal)/4(S_M7_DS [BFSH]) -> "R Stance, Swing, Trans (sagittal)"/16(S_M7_DS)
  R Swing Phase (sagittal)/5(S_M7_Sw [BFSH]) -> "R Stance, Swing, Trans (sagittal)"/17(S_M7_Sw)
  R Swing Phase (sagittal)/6(M8 [RF BFSH]) -> hipM12/1, "R Stance, Swing, Trans (sagittal)"/18(S_M8)
  R Swing Phase (sagittal)/7(M9 [HAM BFSH GAS]) -> hipM11/1, "R Stance, Swing, Trans (sagittal)"/19(S_M9)
  R Swing Phase (sagittal)/8(M10 [HFL GLU VAS]) -> hipM2/1, hipM10/1, "R Stance, Swing, Trans (sagittal)"/20(S_M10)
  Mux1/1 -> [RHSwStim]
  hipM1/1 -> Add3/1
  hipM2/1 -> Add3/2
  Add3/1 -> Mux1/1
  hipM3/1 -> Add2/1
  hipM10/1 -> Add2/2
  Add2/1 -> Mux1/2
  hipM12/1 -> Mux1/3
  hipM11/1 -> Mux1/4
  LL Delay4/1 -> SDelay31/1
  Sum1/1 -> LL Delay4/1
  SDelay31/1 -> R Swing Phase (sagittal)/3(a_tgt)
  [LVceVAS] -> MDelay8/1
  MDelay8/1 -> L Swing Phase (sagittal)/10(VceVAS)
  [RVceVAS] -> MDelay16/1
  MDelay16/1 -> R Swing Phase (sagittal)/10(VceVAS)
  Logical Operator5/1 -> Logical Operator6/2
  Logical Operator6/1 -> R Swing Phase (coronal)/Enable
  [LonR] -> Logical Operator6/1
  [RStance] -> L Stance afferent delay2/1
  L Stance afferent delay2/1 -> Logical Operator5/1, R Stance Phase (coronal)/Enable
  [R_StCtrlPar] -> R Stance Phase (coronal)/1(CtrlPar)
  [R_LHSwStim] -> R Stance Phase (coronal)/4(CSwingStim)
  [R_SwCtrlPar] -> R Swing Phase (coronal)/1(CtrlPar)
  [R_TrCtrlPar] -> "R Stance, Swing, Trans (coronal)"/1(CtrlPar)
  [LonR] -> "R Stance, Swing, Trans (coronal)"/4(ConI)
  [LLLoad] -> SDelay41/1
  SDelay41/1 -> "R Stance, Swing, Trans (coronal)"/6(CLLoad)
  Saturation2/1 -> Demux1/1
  Demux1/2 -> SDelay37/1
  Demux1/1 -> SDelay35/1
  [RLLoad] -> SDelay33/1
  [R_theta_tgt] -> R Stance Phase (coronal)/2(theta_tgt [rad])
  R Swing Phase (coronal)/2(S_M6) -> Sum4/2, "R Stance, Swing, Trans (coronal)"/12(S_M6)
  Sum4/1 -> [R_RHSwStim]
  SDelay33/1 -> "R Stance, Swing, Trans (coronal)"/5(ILLoad)
  R Stance Phase (coronal)/1(S_0_St) -> "R Stance, Swing, Trans (coronal)"/7(S_0_St)
  R Stance Phase (coronal)/3(S_M3 [HAB HAD]) -> "R Stance, Swing, Trans (coronal)"/9(S_M3)
  R Stance Phase (coronal)/4(S_M4 [HAB HAD]) -> "R Stance, Swing, Trans (coronal)"/10(S_M4)
  R Swing Phase (coronal)/1(S_0_Sw) -> Sum4/1, "R Stance, Swing, Trans (coronal)"/11(S_0_Sw)
  [RLceHAD] -> SDelay49/1
  [RLceHAB] -> SDelay34/1
  [RhipR_tgt] -> Sum5/2
  Constant2/1 -> Sum5/3
  [thetaR] -> Sum5/1
  LL Delay7/1 -> SDelay47/1
  SDelay47/1 -> R Stance Phase (coronal)/3(theta dtheta [rad rad/s])
  Mux3/1 -> LL Delay7/1
  LL Delay8/1 -> SDelay48/1
  SDelay48/1 -> R Swing Phase (coronal)/2(R_a_tgt)
  Sum5/1 -> LL Delay8/1
  SDelay49/1 -> R Swing Phase (coronal)/3(LceHAD)
  SDelay34/1 -> R Swing Phase (coronal)/4(LceHAB)
  MDelay21/1 -> "R Stance, Swing, Trans (coronal)"/2(Stance)
  [RStance] -> MDelay21/1
  [LStance] -> MDelay18/1
  MDelay18/1 -> "R Stance, Swing, Trans (coronal)"/3(CStance)
  "R Stance, Swing, Trans (coronal)"/1(S) -> Saturation2/1
  [thetaR] -> Mux3/1
  [dthetaR] -> Mux3/2
  R Stance Phase (coronal)/2(S_M1 [HAB]) -> "R Stance, Swing, Trans (coronal)"/8(S_M1)
  [RFmHAB] -> SDelay38/1
  SDelay38/1 -> R Stance Phase (coronal)/5(FmHAB)
  Logical Operator4/1 -> Logical Operator7/2
  Logical Operator7/1 -> L Swing Phase (coronal)/Enable
  [RonL] -> Logical Operator7/1
  [LStance] -> L Stance afferent delay1/1
  L Stance afferent delay1/1 -> Logical Operator4/1, L Stance Phase (coronal)/Enable
  L GLU Golgi Tendon Organs3/1 -> L Stance Phase (coronal)/2(theta_tgt [rad])
  [R_StCtrlPar] -> L Stance Phase (coronal)/1(CtrlPar)
  [R_RHSwStim] -> L Stance Phase (coronal)/4(CSwingStim)
  [R_SwCtrlPar] -> L Swing Phase (coronal)/1(CtrlPar)
  [R_TrCtrlPar] -> "L Stance, Swing, Trans (coronal)"/1(CtrlPar)
  [RonL] -> "L Stance, Swing, Trans (coronal)"/4(ConI)
  [LStance] -> MDelay22/1
  [RStance] -> MDelay17/1
  [RLLoad] -> SDelay36/1
  SDelay36/1 -> "L Stance, Swing, Trans (coronal)"/6(CLLoad)
  Saturation3/1 -> Demux2/1
  Demux2/2 -> SDelay40/1
  Demux2/1 -> SDelay46/1
  [LLLoad] -> SDelay32/1
  [R_theta_tgt] -> L GLU Golgi Tendon Organs3/1
  Mux5/1 -> L GLU Golgi Tendon Organs1/1
  L Swing Phase (coronal)/2(S_M6 [HAB HAD]) -> Sum2/2, "L Stance, Swing, Trans (coronal)"/12(S_M6)
  Sum2/1 -> [R_LHSwStim]
  SDelay32/1 -> "L Stance, Swing, Trans (coronal)"/5(ILLoad)
  L Stance Phase (coronal)/1(S_0_St) -> "L Stance, Swing, Trans (coronal)"/7(S_0_St)
  L Stance Phase (coronal)/3(S_M3 [HAB HAD]) -> "L Stance, Swing, Trans (coronal)"/9(S_M3)
  L Stance Phase (coronal)/4(S_M4 [HAB HAD]) -> "L Stance, Swing, Trans (coronal)"/10(S_M4)
  L Swing Phase (coronal)/1(S_0_Sw) -> "L Stance, Swing, Trans (coronal)"/11(S_0_Sw), Sum2/1
  [LLceHAD] -> SDelay44/1
  [LLceHAB] -> SDelay45/1
  Constant1/1 -> Sum3/3
  LL Delay6/1 -> SDelay42/1
  SDelay42/1 -> L Stance Phase (coronal)/3(theta dtheta [rad rad/s])
  L GLU Golgi Tendon Organs1/1 -> LL Delay6/1
  LL Delay5/1 -> SDelay43/1
  SDelay43/1 -> L Swing Phase (coronal)/2(R_a_tgt)
  Sum3/1 -> LL Delay5/1
  SDelay44/1 -> L Swing Phase (coronal)/3(LceHAD)
  SDelay45/1 -> L Swing Phase (coronal)/4(LceHAB)
  MDelay22/1 -> "L Stance, Swing, Trans (coronal)"/2(Stance)
  MDelay17/1 -> "L Stance, Swing, Trans (coronal)"/3(CStance)
  SDelay46/1 -> [LStimHAB]
  SDelay40/1 -> [LStimHAD]
  "L Stance, Swing, Trans (coronal)"/1(S) -> Saturation3/1
  [LhipR_tgt] -> Sum3/2
  [thetaR] -> L GLU Golgi Tendon Organs2/1
  L GLU Golgi Tendon Organs2/1 -> Sum3/1
  [thetaR] -> Mux5/1
  [dthetaR] -> Mux5/2
  L Stance Phase (coronal)/2(S_M1 [HAB]) -> "L Stance, Swing, Trans (coronal)"/8(S_M1)
  [LFmHAB] -> SDelay39/1
  SDelay39/1 -> L Stance Phase (coronal)/5(FmHAB)
  SDelay35/1 -> [RStimHAB]
  SDelay37/1 -> [RStimHAD]

== system nms_3Dmodel/etc ==
  note: Fall detection
      | (stop simulation)
  note: Control Parameters
  Abs1 : Abs
  Abs3 : Abs
  Clock : Clock
  Compare To Constant2 : simulink/Logic and Bit Operations/Compare To Constant  relop=>  const=60*pi/180  OutDataTypeStr=boolean
  Compare To Constant6 : simulink/Logic and Bit Operations/Compare To Constant  relop=>  const=60*pi/180  OutDataTypeStr=boolean
  Constant10 : Constant  Value=CtrlPar_Tr
  Constant11 : Constant  Value=CtrlPar_Tr_R
  Constant12 : Constant  Value=CtrlPar_theta0
  Constant2 : Constant  Value=CtrlPar_LL
  Constant3 : Constant  Value=CtrlPar_St_R
  Constant5 : Constant  Value=CtrlPar_St
  Constant6 : Constant  Value=CtrlPar_FP
  Constant7 : Constant  Value=CtrlPar_FP_R
  Constant8 : Constant  Value=CtrlPar_Sw_R
  Constant9 : Constant  Value=CtrlPar_Sw
  Logical Operator2 : Logic  Operator=OR  AllPortsSameDT=off  OutDataTypeStr=boolean
  Stop Simulation : Stop
  To Current Workspace2 : ToWorkspace  VariableName=simout_tEnd  SaveFormat=Structure  SampleTime=-1
      settings: MaxDataPoints=1
  tag scope: FPCtrlPar=global, LLCtrlPar=global, R_FPCtrlPar=global, R_StCtrlPar=global, R_SwCtrlPar=global, R_TrCtrlPar=global, StCtrlPar=global, SwCtrlPar=global, TrCtrlPar=global, theta0=global
  wires:
  [theta] -> Abs3/1
  Abs3/1 -> Compare To Constant2/1
  Compare To Constant2/1 -> Logical Operator2/1
  Logical Operator2/1 -> Stop Simulation/1
  [thetaR] -> Abs1/1
  Abs1/1 -> Compare To Constant6/1
  Compare To Constant6/1 -> Logical Operator2/2
  Constant6/1 -> [FPCtrlPar]
  Constant9/1 -> [SwCtrlPar]
  Constant2/1 -> [LLCtrlPar]
  Constant5/1 -> [StCtrlPar]
  Constant12/1 -> [theta0]
  Constant3/1 -> [R_StCtrlPar]
  Constant7/1 -> [R_FPCtrlPar]
  Constant8/1 -> [R_SwCtrlPar]
  Constant11/1 -> [R_TrCtrlPar]
  Constant10/1 -> [TrCtrlPar]
  Clock/1 -> To Current Workspace2/1

== system nms_3Dmodel/Body Mechanics Layer/LLBall Cnt ==
  note: 3D Ground Interaction Model
  3D Contact : Subsystem
  Body Actuator : mblibv1/Sensors &  Actuators/Body Actuator  UpdateFromCAD=off  PhysicalDomain=Mechanical  PortType=blob  ActuationStyle=Force  AngleUnits=deg  ArcVelocityUnits=deg/s  ArcAccelerationUnits=deg/s^2  CoordPositionUnits=m  VelocityUnits=m/s  AccelerationUnits=m/s^2  ForceUnits=N  TorqueUnits=N*m  ActiveIO=on  Width=3  DialogClass=MechanicalActuatorBlock  ReferenceFrame=Absolute (World)  Angle=off  CoordPosition=on  Force=on  Torque=off
      settings: SourceProductName=Simscape Multibody  SourceProductBaseCode=MS
  Body Sensor : mblibv1/Sensors &  Actuators/Body Sensor  UpdateFromCAD=off  PhysicalDomain=Mechanical  PortType=blob  Muxed=off  Pose=off  Angle=on  AngleUnits=deg  ArcVelocity=off  ArcVelocityUnits=deg/s  ArcAcceleration=off  ArcAccelerationUnits=deg/s^2  CoordPosition=on  CoordPositionUnits=m  Velocity=on  VelocityUnits=m/s  Acceleration=off  AccelerationUnits=m/s^2  Quaternion=on  QuaternionDT=off  QuaternionDDT=off  QuaternionUnits=off  OutputVector=[ 3 3 ]  ActiveIO=on  Width=6  DialogClass=MechanicalSensorBlock  ReferenceFrame=Absolute (World)
      settings: SourceProductName=Simscape Multibody  SourceProductBaseCode=MS
  Demux1 : Demux  Outputs=3
  Mechanical Branching Bar : mblibv1/Utilities/Mechanical Branching Bar  LConnTagsString=_newl0  RConnTagsString=SA0|SA1  UpdateFromCAD=off  DialogClass=MechanicalBranchingBarBlock  NumSAPorts=2
      settings: SourceProductName=Simscape Multibody  SourceProductBaseCode=MS
  Mux : Mux  Inputs=3
  Sum : Sum  Inputs=|+-
  Sum1 : Sum
  Terminator : Terminator
  contact? : simulink/Logic and Bit Operations/Compare To Zero  relop=<=  OutDataTypeStr=boolean
  groundHeight : Constant  Value=0
  nVec : Constant  Value=[0 1 0]
  y : Selector  InputPortWidth=3  IndexOptions=Index vector (dialog)  Indices=2  OutputSizes=1
  F : PMIOPort  Side=Left
  RBallCnt : Outport
  GRF [N N N] : Outport  Port=2
  wires:
  contact?/1 -> 3D Contact/Enable, RBallCnt/1  "cnt"
  Body Sensor/1 -> 3D Contact/3(pVec [m m m]), y/1, Demux1/1  "pos"
  Body Sensor/2 -> 3D Contact/4(vVec [m/s m/s m/s])
  3D Contact/1(FnVec [N N N]) -> Sum1/1
  3D Contact/2(FtVec [N N N]) -> Sum1/2
  Sum1/1 -> GRF [N N N]/1, Body Actuator/1
  Sum/1 -> contact?/1
  y/1 -> Sum/1
  groundHeight/1 -> Mux/2, Sum/2  "EnvHeight"
  Mux/1 -> 3D Contact/1(RefPt [m m m])  "Reference Point RefPt"
  nVec/1 -> 3D Contact/2(nVec [m m m])
  Demux1/1 -> Mux/1
  Demux1/3 -> Mux/3
  Demux1/2 -> Terminator/1
  connections:
  F/RConn1 -- Mechanical Branching Bar/LConn1
  Mechanical Branching Bar/RConn2 -- Body Actuator/RConn1
  Mechanical Branching Bar/RConn1 -- Body Sensor/LConn1

== system nms_3Dmodel/Body Mechanics Layer/LLHeel Cnt ==
  note: 3D Ground Interaction Model
  3D Contact : Subsystem
  Body Actuator : mblibv1/Sensors &  Actuators/Body Actuator  UpdateFromCAD=off  PhysicalDomain=Mechanical  PortType=blob  ActuationStyle=Force  AngleUnits=deg  ArcVelocityUnits=deg/s  ArcAccelerationUnits=deg/s^2  CoordPositionUnits=m  VelocityUnits=m/s  AccelerationUnits=m/s^2  ForceUnits=N  TorqueUnits=N*m  ActiveIO=on  Width=3  DialogClass=MechanicalActuatorBlock  ReferenceFrame=Absolute (World)  Angle=off  CoordPosition=on  Force=on  Torque=off
      settings: SourceProductName=Simscape Multibody  SourceProductBaseCode=MS
  Body Sensor : mblibv1/Sensors &  Actuators/Body Sensor  UpdateFromCAD=off  PhysicalDomain=Mechanical  PortType=blob  Muxed=off  Pose=off  Angle=on  AngleUnits=deg  ArcVelocity=off  ArcVelocityUnits=deg/s  ArcAcceleration=off  ArcAccelerationUnits=deg/s^2  CoordPosition=on  CoordPositionUnits=m  Velocity=on  VelocityUnits=m/s  Acceleration=off  AccelerationUnits=m/s^2  Quaternion=on  QuaternionDT=off  QuaternionDDT=off  QuaternionUnits=off  OutputVector=[ 3 3 ]  ActiveIO=on  Width=6  DialogClass=MechanicalSensorBlock  ReferenceFrame=Absolute (World)
      settings: SourceProductName=Simscape Multibody  SourceProductBaseCode=MS
  Demux1 : Demux  Outputs=3
  Mechanical Branching Bar : mblibv1/Utilities/Mechanical Branching Bar  LConnTagsString=_newl0  RConnTagsString=SA0|SA1  UpdateFromCAD=off  DialogClass=MechanicalBranchingBarBlock  NumSAPorts=2
      settings: SourceProductName=Simscape Multibody  SourceProductBaseCode=MS
  Mux : Mux  Inputs=3
  Sum : Sum  Inputs=|+-
  Sum1 : Sum
  Terminator : Terminator
  contact? : simulink/Logic and Bit Operations/Compare To Zero  relop=<=  OutDataTypeStr=boolean
  groundHeight : Constant  Value=0
  nVec : Constant  Value=[0 1 0]
  y : Selector  InputPortWidth=3  IndexOptions=Index vector (dialog)  Indices=2  OutputSizes=1
  F : PMIOPort  Side=Left
  RBallCnt : Outport
  GRF [N N N] : Outport  Port=2
  wires:
  contact?/1 -> 3D Contact/Enable, RBallCnt/1  "cnt"
  Body Sensor/1 -> 3D Contact/3(pVec [m m m]), y/1, Demux1/1  "pos"
  Body Sensor/2 -> 3D Contact/4(vVec [m/s m/s m/s])
  3D Contact/1(FnVec [N N N]) -> Sum1/1
  3D Contact/2(FtVec [N N N]) -> Sum1/2
  Sum1/1 -> GRF [N N N]/1, Body Actuator/1
  Sum/1 -> contact?/1
  y/1 -> Sum/1
  groundHeight/1 -> Mux/2, Sum/2  "EnvHeight"
  Mux/1 -> 3D Contact/1(RefPt [m m m])  "Reference Point RefPt"
  nVec/1 -> 3D Contact/2(nVec [m m m])
  Demux1/1 -> Mux/1
  Demux1/3 -> Mux/3
  Demux1/2 -> Terminator/1
  connections:
  F/RConn1 -- Mechanical Branching Bar/LConn1
  Mechanical Branching Bar/RConn2 -- Body Actuator/RConn1
  Mechanical Branching Bar/RConn1 -- Body Sensor/LConn1
